simulink model "DC_motor_modell"  (R2020b)
settings: Solver=VariableStepAuto  StartTime=0.0  StopTime=100  RelTol=1e-3
settings Model: Creator=alfac  LastModifiedBy=Legion1
settings DataIOCC: ReturnWorkspaceOutputs=off
settings DebuggingCC: ArithmeticOperatorsInVariantConditions=warning
settings SFSimCC: SimUseLocalCustomCode=off  CustomCodeUndefinedFunction=UseInterfaceOnly
settings RTWCC: RTWUseLocalCustomCode=off

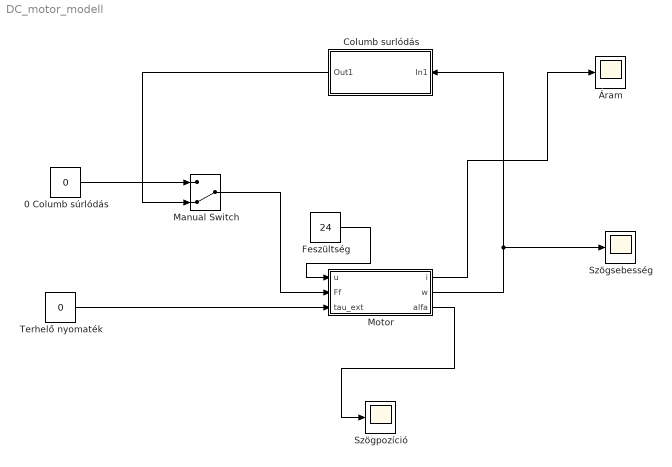
== system DC_motor_modell ==
  0 Columb súrlódás : Constant  Value=0
  Columb surlódás : Subsystem  mask{c2=38.2 *0.001, i_no_load=74 *0.001}
  Feszültség : Constant  Value=24
  Manual Switch : ManualSwitch  CurrentSetting=0
  Motor : Subsystem  mask{R=7.13, L=1.05 * 0.001, c1=1/26.16, c2=38.2 *10^-7, Jr=41.9}
  Szögpozíció : Scope
  Szögsebesség : Scope
  Terhelő nyomaték : Constant  Value=0
  Áram : Scope
  wires:
  Motor/1(i) -> Áram/1
  Motor/2(w) -> Columb surlódás/1(In1), Szögsebesség/1
  Motor/3(alfa) -> Szögpozíció/1
  Feszültség/1 -> Motor/1(u)
  Terhelő nyomaték/1 -> Motor/3(tau_ext)
  Columb surlódás/1(Out1) -> Manual Switch/2
  Manual Switch/1 -> Motor/2(Ff)
  0 Columb súrlódás/1 -> Manual Switch/1

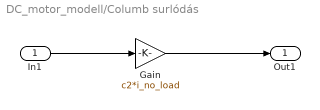
== system DC_motor_modell/Columb surlódás ==
  In1 : Inport
  Gain : Gain  Gain=c2*i_no_load
  Out1 : Outport  VectorParamsAs1DForOutWhenUnconnected=off
  wires:
  In1/1 -> Gain/1
  Gain/1 -> Out1/1

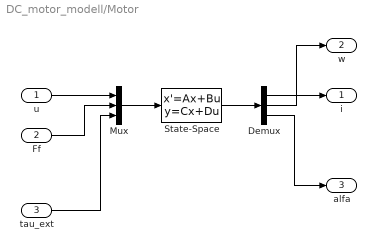
== system DC_motor_modell/Motor ==
  u : Inport  OutDataTypeStr=double
  Ff : Inport  Port=2  OutDataTypeStr=double
  tau_ext : Inport  Port=3  OutDataTypeStr=double
  Demux : Demux  Outputs=[1;1;1]
  Mux : Mux  Inputs=3
  State-Space : StateSpace  A="[-R/L    -c1/L    0; c2/Jr   0    0;    0 1 0]"  B=[1/L 0 0; 0 -1/Jr -1/Jr; 0 0 0]  C=[1 0 0; 0 1 0; 0 0 1]  D=[0 0 0; 0 0 0; 0 0 0]  InitialCondition=[0 0 0]
  i : Outport  PortDimensions=1  SampleTime=1  VectorParamsAs1DForOutWhenUnconnected=off
  w : Outport  Port=2  PortDimensions=1  SampleTime=1  VectorParamsAs1DForOutWhenUnconnected=off
  alfa : Outport  Port=3  PortDimensions=1  SampleTime=1  VectorParamsAs1DForOutWhenUnconnected=off
  wires:
  u/1 -> Mux/1
  Ff/1 -> Mux/2
  tau_ext/1 -> Mux/3
  Mux/1 -> State-Space/1
  State-Space/1 -> Demux/1
  Demux/3 -> alfa/1
  Demux/2 -> w/1
  Demux/1 -> i/1
